simulink model "gm_smartCart4_1_work"  (R2016a)
settings: Solver=FixedStepDiscrete  StartTime=0.0  StopTime=100000  FixedStep=1  RelTol=1e-3
libraries: simulink x103, hdlsllib x73
(part 3 of 3)

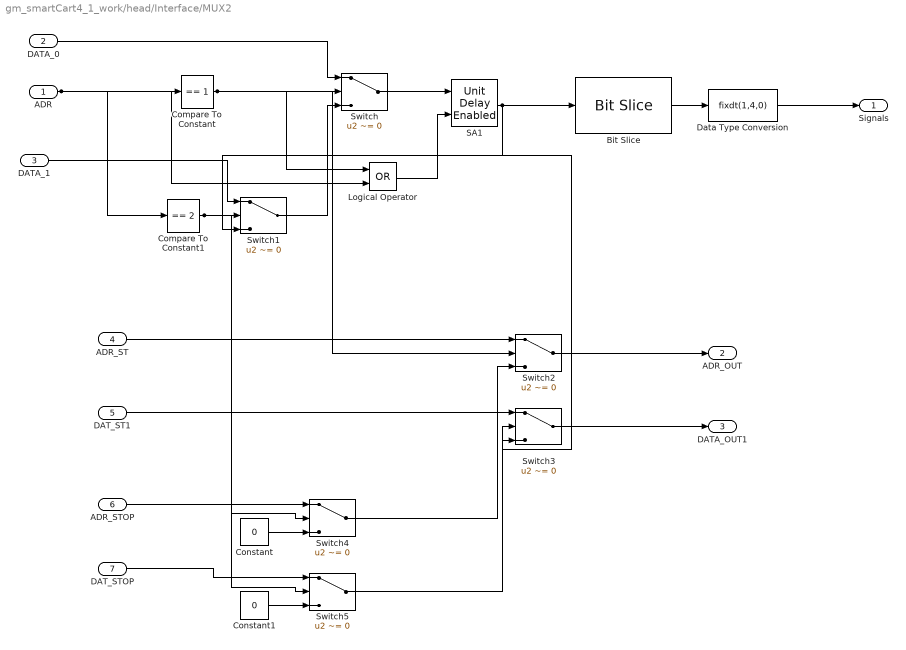
== system gm_smartCart4_1_work/head/Interface/MUX2 ==
  ADR : Inport  OutDataTypeStr=uint8  SampleTime=1
  DATA_0 : Inport  Port=2  OutDataTypeStr=uint8  SampleTime=1
  DATA_1 : Inport  Port=3  OutDataTypeStr=uint8  SampleTime=1
  ADR_ST : Inport  Port=4  OutDataTypeStr=uint8  SampleTime=1
  DAT_ST1 : Inport  Port=5  OutDataTypeStr=uint8  SampleTime=1
  ADR_STOP : Inport  Port=6  OutDataTypeStr=uint8  SampleTime=1
  DAT_STOP : Inport  Port=7  OutDataTypeStr=uint8  SampleTime=1
  Bit Slice : hdlsllib/HDL Operations/Bit Slice  lidx=4  ridx=0
  Compare To Constant : simulink/Logic and Bit Operations/Compare To Constant  relop===  const=1  OutDataTypeStr=boolean
  Compare To Constant1 : simulink/Logic and Bit Operations/Compare To Constant  relop===  const=2  OutDataTypeStr=boolean
  Constant : Constant  Value=0  OutDataTypeStr=boolean
  Constant1 : Constant  Value=0  OutDataTypeStr=boolean
  Data Type Conversion : DataTypeConversion  OutDataTypeStr=fixdt(1,4,0)
  Logical Operator : Logic  Operator=OR  AllPortsSameDT=off  OutDataTypeStr=boolean
  SA1 : simulink/Additional Math & Discrete/Additional Discrete/Unit Delay Enabled  vinit=0  tsamp=-1
  Switch{,1..5} (6 alike) : Switch  Criteria=u2 ~= 0  OutDataTypeStr=uint8
  Signals : Outport  OutDataTypeStr=fixdt(1,4,0)
  ADR_OUT : Outport  Port=2  OutDataTypeStr=uint8
  DATA_OUT1 : Outport  Port=3  OutDataTypeStr=uint8
  wires:
  ADR/1 -> Logical Operator/2, Compare To Constant1/1, Compare To Constant/1
  DATA_0/1 -> Switch/1
  DATA_1/1 -> Switch1/1
  ADR_ST/1 -> Switch2/1
  DAT_ST1/1 -> Switch3/1
  ADR_STOP/1 -> Switch4/1
  DAT_STOP/1 -> Switch5/1
  Bit Slice/1 -> Data Type Conversion/1
  Compare To Constant/1 -> Switch3/2, Switch2/2, Switch/2, Logical Operator/1
  Compare To Constant1/1 -> Switch5/2, Switch4/2, Switch1/2
  Constant/1 -> Switch4/3
  Constant1/1 -> Switch5/3
  Data Type Conversion/1 -> Signals/1
  Logical Operator/1 -> SA1/2
  SA1/1 -> Switch1/3, Bit Slice/1
  Switch/1 -> SA1/1
  Switch1/1 -> Switch/3
  Switch2/1 -> ADR_OUT/1
  Switch3/1 -> DATA_OUT1/1
  Switch4/1 -> Switch2/3
  Switch5/1 -> Switch3/3

== system gm_smartCart4_1_work/head/Interface/Swith_signal2 ==
  Adr : Inport  OutDataTypeStr=uint8  SampleTime=1
  Data : Inport  Port=2  OutDataTypeStr=uint8  SampleTime=1
  Compare To Constant : simulink/Logic and Bit Operations/Compare To Constant  relop===  const=2  OutDataTypeStr=boolean
  SA1 : simulink/Additional Math & Discrete/Additional Discrete/Unit Delay Enabled  vinit=0  tsamp=-1
  OutAddr : Outport  OutDataTypeStr=uint8
  wires:
  Adr/1 -> Compare To Constant/1
  Data/1 -> SA1/1
  Compare To Constant/1 -> SA1/2
  SA1/1 -> OutAddr/1

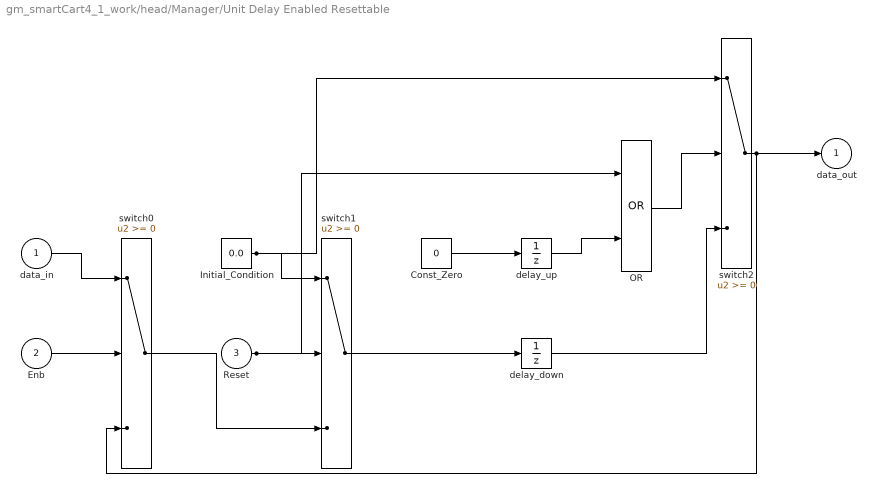
== system gm_smartCart4_1_work/head/Manager/Unit Delay Enabled Resettable ==
  data_in : Inport
  Enb : Inport  Port=2
  Reset : Inport  Port=3
  Const_Zero : Constant  Value=0  OutDataTypeStr=boolean
  Initial_Condition : Constant  Value=0.0  OutDataTypeStr=Inherit: Inherit via back propagation
  OR : Logic  Operator=OR
  delay_down : UnitDelay  SampleTime=-1
  delay_up : UnitDelay  InitialCondition=1  SampleTime=-1
  switch0 : Switch  SaturateOnIntegerOverflow=on  InputSameDT=on
  switch1 : Switch  SaturateOnIntegerOverflow=on  InputSameDT=on
  switch2 : Switch  SaturateOnIntegerOverflow=on  InputSameDT=on
  data_out : Outport
  wires:
  data_in/1 -> switch0/1
  Enb/1 -> switch0/2
  switch2/1 -> switch0/3, data_out/1
  Initial_Condition/1 -> switch1/1, switch2/1
  Reset/1 -> switch1/2, OR/1
  switch0/1 -> switch1/3
  Const_Zero/1 -> delay_up/1
  switch1/1 -> delay_down/1
  delay_up/1 -> OR/2
  OR/1 -> switch2/2
  delay_down/1 -> switch2/3

== system gm_smartCart4_1_work/head/Manager/Unit Delay Enabled Resettable1 ==
  data_in : Inport
  Enb : Inport  Port=2
  Reset : Inport  Port=3
  Const_Zero : Constant  Value=0  OutDataTypeStr=boolean
  Initial_Condition : Constant  Value=0.0  OutDataTypeStr=Inherit: Inherit via back propagation
  OR : Logic  Operator=OR
  delay_down : UnitDelay  SampleTime=-1
  delay_up : UnitDelay  InitialCondition=1  SampleTime=-1
  switch0 : Switch  SaturateOnIntegerOverflow=on  InputSameDT=on
  switch1 : Switch  SaturateOnIntegerOverflow=on  InputSameDT=on
  switch2 : Switch  SaturateOnIntegerOverflow=on  InputSameDT=on
  data_out : Outport
  wires:
  data_in/1 -> switch0/1
  Enb/1 -> switch0/2
  switch2/1 -> switch0/3, data_out/1
  Initial_Condition/1 -> switch1/1, switch2/1
  Reset/1 -> switch1/2, OR/1
  switch0/1 -> switch1/3
  Const_Zero/1 -> delay_up/1
  switch1/1 -> delay_down/1
  delay_up/1 -> OR/2
  OR/1 -> switch2/2
  delay_down/1 -> switch2/3

== system gm_smartCart4_1_work/head/Manager/Unit Delay Enabled Resettable10 ==
  data_in : Inport
  Enb : Inport  Port=2
  Reset : Inport  Port=3
  Const_Zero : Constant  Value=0  OutDataTypeStr=boolean
  Initial_Condition : Constant  Value=0.0  OutDataTypeStr=Inherit: Inherit via back propagation
  OR : Logic  Operator=OR
  delay_down : UnitDelay  SampleTime=-1
  delay_up : UnitDelay  InitialCondition=1  SampleTime=-1
  switch0 : Switch  SaturateOnIntegerOverflow=on  InputSameDT=on
  switch1 : Switch  SaturateOnIntegerOverflow=on  InputSameDT=on
  switch2 : Switch  SaturateOnIntegerOverflow=on  InputSameDT=on
  data_out : Outport
  wires:
  data_in/1 -> switch0/1
  Enb/1 -> switch0/2
  switch2/1 -> switch0/3, data_out/1
  Initial_Condition/1 -> switch1/1, switch2/1
  Reset/1 -> switch1/2, OR/1
  switch0/1 -> switch1/3
  Const_Zero/1 -> delay_up/1
  switch1/1 -> delay_down/1
  delay_up/1 -> OR/2
  OR/1 -> switch2/2
  delay_down/1 -> switch2/3

== system gm_smartCart4_1_work/head/Manager/Unit Delay Enabled Resettable11 ==
  data_in : Inport
  Enb : Inport  Port=2
  Reset : Inport  Port=3
  Const_Zero : Constant  Value=0  OutDataTypeStr=boolean
  Initial_Condition : Constant  Value=0.0  OutDataTypeStr=Inherit: Inherit via back propagation
  OR : Logic  Operator=OR
  delay_down : UnitDelay  SampleTime=-1
  delay_up : UnitDelay  InitialCondition=1  SampleTime=-1
  switch0 : Switch  SaturateOnIntegerOverflow=on  InputSameDT=on
  switch1 : Switch  SaturateOnIntegerOverflow=on  InputSameDT=on
  switch2 : Switch  SaturateOnIntegerOverflow=on  InputSameDT=on
  data_out : Outport
  wires:
  data_in/1 -> switch0/1
  Enb/1 -> switch0/2
  switch2/1 -> switch0/3, data_out/1
  Initial_Condition/1 -> switch1/1, switch2/1
  Reset/1 -> switch1/2, OR/1
  switch0/1 -> switch1/3
  Const_Zero/1 -> delay_up/1
  switch1/1 -> delay_down/1
  delay_up/1 -> OR/2
  OR/1 -> switch2/2
  delay_down/1 -> switch2/3

== system gm_smartCart4_1_work/head/Manager/Unit Delay Enabled Resettable12 ==
  data_in : Inport
  Enb : Inport  Port=2
  Reset : Inport  Port=3
  Const_Zero : Constant  Value=0  OutDataTypeStr=boolean
  Initial_Condition : Constant  Value=0.0  OutDataTypeStr=Inherit: Inherit via back propagation
  OR : Logic  Operator=OR
  delay_down : UnitDelay  SampleTime=-1
  delay_up : UnitDelay  InitialCondition=1  SampleTime=-1
  switch0 : Switch  SaturateOnIntegerOverflow=on  InputSameDT=on
  switch1 : Switch  SaturateOnIntegerOverflow=on  InputSameDT=on
  switch2 : Switch  SaturateOnIntegerOverflow=on  InputSameDT=on
  data_out : Outport
  wires:
  data_in/1 -> switch0/1
  Enb/1 -> switch0/2
  switch2/1 -> switch0/3, data_out/1
  Initial_Condition/1 -> switch1/1, switch2/1
  Reset/1 -> switch1/2, OR/1
  switch0/1 -> switch1/3
  Const_Zero/1 -> delay_up/1
  switch1/1 -> delay_down/1
  delay_up/1 -> OR/2
  OR/1 -> switch2/2
  delay_down/1 -> switch2/3

== system gm_smartCart4_1_work/head/Manager/Unit Delay Enabled Resettable13 ==
  data_in : Inport
  Enb : Inport  Port=2
  Reset : Inport  Port=3
  Const_Zero : Constant  Value=0  OutDataTypeStr=boolean
  Initial_Condition : Constant  Value=0.0  OutDataTypeStr=Inherit: Inherit via back propagation
  OR : Logic  Operator=OR
  delay_down : UnitDelay  SampleTime=-1
  delay_up : UnitDelay  InitialCondition=1  SampleTime=-1
  switch0 : Switch  SaturateOnIntegerOverflow=on  InputSameDT=on
  switch1 : Switch  SaturateOnIntegerOverflow=on  InputSameDT=on
  switch2 : Switch  SaturateOnIntegerOverflow=on  InputSameDT=on
  data_out : Outport
  wires:
  data_in/1 -> switch0/1
  Enb/1 -> switch0/2
  switch2/1 -> switch0/3, data_out/1
  Initial_Condition/1 -> switch1/1, switch2/1
  Reset/1 -> switch1/2, OR/1
  switch0/1 -> switch1/3
  Const_Zero/1 -> delay_up/1
  switch1/1 -> delay_down/1
  delay_up/1 -> OR/2
  OR/1 -> switch2/2
  delay_down/1 -> switch2/3

== system gm_smartCart4_1_work/head/Manager/Unit Delay Enabled Resettable14 ==
  data_in : Inport
  Enb : Inport  Port=2
  Reset : Inport  Port=3
  Const_Zero : Constant  Value=0  OutDataTypeStr=boolean
  Initial_Condition : Constant  Value=0  OutDataTypeStr=Inherit: Inherit via back propagation
  OR : Logic  Operator=OR
  delay_down : UnitDelay  SampleTime=-1
  delay_up : UnitDelay  InitialCondition=1  SampleTime=-1
  switch0 : Switch  SaturateOnIntegerOverflow=on  InputSameDT=on
  switch1 : Switch  SaturateOnIntegerOverflow=on  InputSameDT=on
  switch2 : Switch  SaturateOnIntegerOverflow=on  InputSameDT=on
  data_out : Outport
  wires:
  data_in/1 -> switch0/1
  Enb/1 -> switch0/2
  switch2/1 -> switch0/3, data_out/1
  Initial_Condition/1 -> switch1/1, switch2/1
  Reset/1 -> switch1/2, OR/1
  switch0/1 -> switch1/3
  Const_Zero/1 -> delay_up/1
  switch1/1 -> delay_down/1
  delay_up/1 -> OR/2
  OR/1 -> switch2/2
  delay_down/1 -> switch2/3

== system gm_smartCart4_1_work/head/Manager/Unit Delay Enabled Resettable15 ==
  data_in : Inport
  Enb : Inport  Port=2
  Reset : Inport  Port=3
  Const_Zero : Constant  Value=0  OutDataTypeStr=boolean
  Initial_Condition : Constant  Value=0.0  OutDataTypeStr=Inherit: Inherit via back propagation
  OR : Logic  Operator=OR
  delay_down : UnitDelay  SampleTime=-1
  delay_up : UnitDelay  InitialCondition=1  SampleTime=-1
  switch0 : Switch  SaturateOnIntegerOverflow=on  InputSameDT=on
  switch1 : Switch  SaturateOnIntegerOverflow=on  InputSameDT=on
  switch2 : Switch  SaturateOnIntegerOverflow=on  InputSameDT=on
  data_out : Outport
  wires:
  data_in/1 -> switch0/1
  Enb/1 -> switch0/2
  switch2/1 -> switch0/3, data_out/1
  Initial_Condition/1 -> switch1/1, switch2/1
  Reset/1 -> switch1/2, OR/1
  switch0/1 -> switch1/3
  Const_Zero/1 -> delay_up/1
  switch1/1 -> delay_down/1
  delay_up/1 -> OR/2
  OR/1 -> switch2/2
  delay_down/1 -> switch2/3

== system gm_smartCart4_1_work/head/Manager/Unit Delay Enabled Resettable16 ==
  data_in : Inport
  Enb : Inport  Port=2
  Reset : Inport  Port=3
  Const_Zero : Constant  Value=0  OutDataTypeStr=boolean
  Initial_Condition : Constant  Value=0  OutDataTypeStr=Inherit: Inherit via back propagation
  OR : Logic  Operator=OR
  delay_down : UnitDelay  SampleTime=-1
  delay_up : UnitDelay  InitialCondition=1  SampleTime=-1
  switch0 : Switch  SaturateOnIntegerOverflow=on  InputSameDT=on
  switch1 : Switch  SaturateOnIntegerOverflow=on  InputSameDT=on
  switch2 : Switch  SaturateOnIntegerOverflow=on  InputSameDT=on
  data_out : Outport
  wires:
  data_in/1 -> switch0/1
  Enb/1 -> switch0/2
  switch2/1 -> switch0/3, data_out/1
  Initial_Condition/1 -> switch1/1, switch2/1
  Reset/1 -> switch1/2, OR/1
  switch0/1 -> switch1/3
  Const_Zero/1 -> delay_up/1
  switch1/1 -> delay_down/1
  delay_up/1 -> OR/2
  OR/1 -> switch2/2
  delay_down/1 -> switch2/3

== system gm_smartCart4_1_work/head/Manager/Unit Delay Enabled Resettable17 ==
  data_in : Inport
  Enb : Inport  Port=2
  Reset : Inport  Port=3
  Const_Zero : Constant  Value=0  OutDataTypeStr=boolean
  Initial_Condition : Constant  Value=0  OutDataTypeStr=Inherit: Inherit via back propagation
  OR : Logic  Operator=OR
  delay_down : UnitDelay  SampleTime=-1
  delay_up : UnitDelay  InitialCondition=1  SampleTime=-1
  switch0 : Switch  SaturateOnIntegerOverflow=on  InputSameDT=on
  switch1 : Switch  SaturateOnIntegerOverflow=on  InputSameDT=on
  switch2 : Switch  SaturateOnIntegerOverflow=on  InputSameDT=on
  data_out : Outport
  wires:
  data_in/1 -> switch0/1
  Enb/1 -> switch0/2
  switch2/1 -> switch0/3, data_out/1
  Initial_Condition/1 -> switch1/1, switch2/1
  Reset/1 -> switch1/2, OR/1
  switch0/1 -> switch1/3
  Const_Zero/1 -> delay_up/1
  switch1/1 -> delay_down/1
  delay_up/1 -> OR/2
  OR/1 -> switch2/2
  delay_down/1 -> switch2/3

== system gm_smartCart4_1_work/head/Manager/Unit Delay Enabled Resettable18 ==
  data_in : Inport
  Enb : Inport  Port=2
  Reset : Inport  Port=3
  Const_Zero : Constant  Value=0  OutDataTypeStr=boolean
  Initial_Condition : Constant  Value=0  OutDataTypeStr=Inherit: Inherit via back propagation
  OR : Logic  Operator=OR
  delay_down : UnitDelay  SampleTime=-1
  delay_up : UnitDelay  InitialCondition=1  SampleTime=-1
  switch0 : Switch  SaturateOnIntegerOverflow=on  InputSameDT=on
  switch1 : Switch  SaturateOnIntegerOverflow=on  InputSameDT=on
  switch2 : Switch  SaturateOnIntegerOverflow=on  InputSameDT=on
  data_out : Outport
  wires:
  data_in/1 -> switch0/1
  Enb/1 -> switch0/2
  switch2/1 -> switch0/3, data_out/1
  Initial_Condition/1 -> switch1/1, switch2/1
  Reset/1 -> switch1/2, OR/1
  switch0/1 -> switch1/3
  Const_Zero/1 -> delay_up/1
  switch1/1 -> delay_down/1
  delay_up/1 -> OR/2
  OR/1 -> switch2/2
  delay_down/1 -> switch2/3

== system gm_smartCart4_1_work/head/Manager/Unit Delay Enabled Resettable19 ==
  data_in : Inport
  Enb : Inport  Port=2
  Reset : Inport  Port=3
  Const_Zero : Constant  Value=0  OutDataTypeStr=boolean
  Initial_Condition : Constant  Value=0  OutDataTypeStr=Inherit: Inherit via back propagation
  OR : Logic  Operator=OR
  delay_down : UnitDelay  SampleTime=-1
  delay_up : UnitDelay  InitialCondition=1  SampleTime=-1
  switch0 : Switch  SaturateOnIntegerOverflow=on  InputSameDT=on
  switch1 : Switch  SaturateOnIntegerOverflow=on  InputSameDT=on
  switch2 : Switch  SaturateOnIntegerOverflow=on  InputSameDT=on
  data_out : Outport
  wires:
  data_in/1 -> switch0/1
  Enb/1 -> switch0/2
  switch2/1 -> switch0/3, data_out/1
  Initial_Condition/1 -> switch1/1, switch2/1
  Reset/1 -> switch1/2, OR/1
  switch0/1 -> switch1/3
  Const_Zero/1 -> delay_up/1
  switch1/1 -> delay_down/1
  delay_up/1 -> OR/2
  OR/1 -> switch2/2
  delay_down/1 -> switch2/3

== system gm_smartCart4_1_work/head/Manager/Unit Delay Enabled Resettable2 ==
  data_in : Inport
  Enb : Inport  Port=2
  Reset : Inport  Port=3
  Const_Zero : Constant  Value=0  OutDataTypeStr=boolean
  Initial_Condition : Constant  Value=0.0  OutDataTypeStr=Inherit: Inherit via back propagation
  OR : Logic  Operator=OR
  delay_down : UnitDelay  SampleTime=-1
  delay_up : UnitDelay  InitialCondition=1  SampleTime=-1
  switch0 : Switch  SaturateOnIntegerOverflow=on  InputSameDT=on
  switch1 : Switch  SaturateOnIntegerOverflow=on  InputSameDT=on
  switch2 : Switch  SaturateOnIntegerOverflow=on  InputSameDT=on
  data_out : Outport
  wires:
  data_in/1 -> switch0/1
  Enb/1 -> switch0/2
  switch2/1 -> switch0/3, data_out/1
  Initial_Condition/1 -> switch1/1, switch2/1
  Reset/1 -> switch1/2, OR/1
  switch0/1 -> switch1/3
  Const_Zero/1 -> delay_up/1
  switch1/1 -> delay_down/1
  delay_up/1 -> OR/2
  OR/1 -> switch2/2
  delay_down/1 -> switch2/3

== system gm_smartCart4_1_work/head/Manager/Unit Delay Enabled Resettable20 ==
  data_in : Inport
  Enb : Inport  Port=2
  Reset : Inport  Port=3
  Const_Zero : Constant  Value=0  OutDataTypeStr=boolean
  Initial_Condition : Constant  Value=0  OutDataTypeStr=Inherit: Inherit via back propagation
  OR : Logic  Operator=OR
  delay_down : UnitDelay  SampleTime=-1
  delay_up : UnitDelay  InitialCondition=1  SampleTime=-1
  switch0 : Switch  SaturateOnIntegerOverflow=on  InputSameDT=on
  switch1 : Switch  SaturateOnIntegerOverflow=on  InputSameDT=on
  switch2 : Switch  SaturateOnIntegerOverflow=on  InputSameDT=on
  data_out : Outport
  wires:
  data_in/1 -> switch0/1
  Enb/1 -> switch0/2
  switch2/1 -> switch0/3, data_out/1
  Initial_Condition/1 -> switch1/1, switch2/1
  Reset/1 -> switch1/2, OR/1
  switch0/1 -> switch1/3
  Const_Zero/1 -> delay_up/1
  switch1/1 -> delay_down/1
  delay_up/1 -> OR/2
  OR/1 -> switch2/2
  delay_down/1 -> switch2/3

== system gm_smartCart4_1_work/head/Manager/Unit Delay Enabled Resettable21 ==
  data_in : Inport
  Enb : Inport  Port=2
  Reset : Inport  Port=3
  Const_Zero : Constant  Value=0  OutDataTypeStr=boolean
  Initial_Condition : Constant  Value=0  OutDataTypeStr=Inherit: Inherit via back propagation
  OR : Logic  Operator=OR
  delay_down : UnitDelay  SampleTime=-1
  delay_up : UnitDelay  InitialCondition=1  SampleTime=-1
  switch0 : Switch  SaturateOnIntegerOverflow=on  InputSameDT=on
  switch1 : Switch  SaturateOnIntegerOverflow=on  InputSameDT=on
  switch2 : Switch  SaturateOnIntegerOverflow=on  InputSameDT=on
  data_out : Outport
  wires:
  data_in/1 -> switch0/1
  Enb/1 -> switch0/2
  switch2/1 -> switch0/3, data_out/1
  Initial_Condition/1 -> switch1/1, switch2/1
  Reset/1 -> switch1/2, OR/1
  switch0/1 -> switch1/3
  Const_Zero/1 -> delay_up/1
  switch1/1 -> delay_down/1
  delay_up/1 -> OR/2
  OR/1 -> switch2/2
  delay_down/1 -> switch2/3

== system gm_smartCart4_1_work/head/Manager/Unit Delay Enabled Resettable22 ==
  data_in : Inport
  Enb : Inport  Port=2
  Reset : Inport  Port=3
  Const_Zero : Constant  Value=0  OutDataTypeStr=boolean
  Initial_Condition : Constant  Value=0  OutDataTypeStr=Inherit: Inherit via back propagation
  OR : Logic  Operator=OR
  delay_down : UnitDelay  SampleTime=-1
  delay_up : UnitDelay  InitialCondition=1  SampleTime=-1
  switch0 : Switch  SaturateOnIntegerOverflow=on  InputSameDT=on
  switch1 : Switch  SaturateOnIntegerOverflow=on  InputSameDT=on
  switch2 : Switch  SaturateOnIntegerOverflow=on  InputSameDT=on
  data_out : Outport
  wires:
  data_in/1 -> switch0/1
  Enb/1 -> switch0/2
  switch2/1 -> switch0/3, data_out/1
  Initial_Condition/1 -> switch1/1, switch2/1
  Reset/1 -> switch1/2, OR/1
  switch0/1 -> switch1/3
  Const_Zero/1 -> delay_up/1
  switch1/1 -> delay_down/1
  delay_up/1 -> OR/2
  OR/1 -> switch2/2
  delay_down/1 -> switch2/3

== system gm_smartCart4_1_work/head/Manager/Unit Delay Enabled Resettable23 ==
  data_in : Inport
  Enb : Inport  Port=2
  Reset : Inport  Port=3
  Const_Zero : Constant  Value=0  OutDataTypeStr=boolean
  Initial_Condition : Constant  Value=0  OutDataTypeStr=Inherit: Inherit via back propagation
  OR : Logic  Operator=OR
  delay_down : UnitDelay  SampleTime=-1
  delay_up : UnitDelay  InitialCondition=1  SampleTime=-1
  switch0 : Switch  SaturateOnIntegerOverflow=on  InputSameDT=on
  switch1 : Switch  SaturateOnIntegerOverflow=on  InputSameDT=on
  switch2 : Switch  SaturateOnIntegerOverflow=on  InputSameDT=on
  data_out : Outport
  wires:
  data_in/1 -> switch0/1
  Enb/1 -> switch0/2
  switch2/1 -> switch0/3, data_out/1
  Initial_Condition/1 -> switch1/1, switch2/1
  Reset/1 -> switch1/2, OR/1
  switch0/1 -> switch1/3
  Const_Zero/1 -> delay_up/1
  switch1/1 -> delay_down/1
  delay_up/1 -> OR/2
  OR/1 -> switch2/2
  delay_down/1 -> switch2/3

== system gm_smartCart4_1_work/head/Manager/Unit Delay Enabled Resettable24 ==
  data_in : Inport
  Enb : Inport  Port=2
  Reset : Inport  Port=3
  Const_Zero : Constant  Value=0  OutDataTypeStr=boolean
  Initial_Condition : Constant  Value=0  OutDataTypeStr=Inherit: Inherit via back propagation
  OR : Logic  Operator=OR
  delay_down : UnitDelay  SampleTime=-1
  delay_up : UnitDelay  InitialCondition=1  SampleTime=-1
  switch0 : Switch  SaturateOnIntegerOverflow=on  InputSameDT=on
  switch1 : Switch  SaturateOnIntegerOverflow=on  InputSameDT=on
  switch2 : Switch  SaturateOnIntegerOverflow=on  InputSameDT=on
  data_out : Outport
  wires:
  data_in/1 -> switch0/1
  Enb/1 -> switch0/2
  switch2/1 -> switch0/3, data_out/1
  Initial_Condition/1 -> switch1/1, switch2/1
  Reset/1 -> switch1/2, OR/1
  switch0/1 -> switch1/3
  Const_Zero/1 -> delay_up/1
  switch1/1 -> delay_down/1
  delay_up/1 -> OR/2
  OR/1 -> switch2/2
  delay_down/1 -> switch2/3

== system gm_smartCart4_1_work/head/Manager/Unit Delay Enabled Resettable26 ==
  data_in : Inport
  Enb : Inport  Port=2
  Reset : Inport  Port=3
  Const_Zero : Constant  Value=0  OutDataTypeStr=boolean
  Initial_Condition : Constant  Value=0  OutDataTypeStr=Inherit: Inherit via back propagation
  OR : Logic  Operator=OR
  delay_down : UnitDelay  SampleTime=-1
  delay_up : UnitDelay  InitialCondition=1  SampleTime=-1
  switch0 : Switch  SaturateOnIntegerOverflow=on  InputSameDT=on
  switch1 : Switch  SaturateOnIntegerOverflow=on  InputSameDT=on
  switch2 : Switch  SaturateOnIntegerOverflow=on  InputSameDT=on
  data_out : Outport
  wires:
  data_in/1 -> switch0/1
  Enb/1 -> switch0/2
  switch2/1 -> switch0/3, data_out/1
  Initial_Condition/1 -> switch1/1, switch2/1
  Reset/1 -> switch1/2, OR/1
  switch0/1 -> switch1/3
  Const_Zero/1 -> delay_up/1
  switch1/1 -> delay_down/1
  delay_up/1 -> OR/2
  OR/1 -> switch2/2
  delay_down/1 -> switch2/3

== system gm_smartCart4_1_work/head/Manager/Unit Delay Enabled Resettable28 ==
  data_in : Inport
  Enb : Inport  Port=2
  Reset : Inport  Port=3
  Const_Zero : Constant  Value=0  OutDataTypeStr=boolean
  Initial_Condition : Constant  Value=0  OutDataTypeStr=Inherit: Inherit via back propagation
  OR : Logic  Operator=OR
  delay_down : UnitDelay  SampleTime=-1
  delay_up : UnitDelay  InitialCondition=1  SampleTime=-1
  switch0 : Switch  SaturateOnIntegerOverflow=on  InputSameDT=on
  switch1 : Switch  SaturateOnIntegerOverflow=on  InputSameDT=on
  switch2 : Switch  SaturateOnIntegerOverflow=on  InputSameDT=on
  data_out : Outport
  wires:
  data_in/1 -> switch0/1
  Enb/1 -> switch0/2
  switch2/1 -> switch0/3, data_out/1
  Initial_Condition/1 -> switch1/1, switch2/1
  Reset/1 -> switch1/2, OR/1
  switch0/1 -> switch1/3
  Const_Zero/1 -> delay_up/1
  switch1/1 -> delay_down/1
  delay_up/1 -> OR/2
  OR/1 -> switch2/2
  delay_down/1 -> switch2/3

== system gm_smartCart4_1_work/head/Manager/Unit Delay Enabled Resettable3 ==
  data_in : Inport
  Enb : Inport  Port=2
  Reset : Inport  Port=3
  Const_Zero : Constant  Value=0  OutDataTypeStr=boolean
  Initial_Condition : Constant  Value=0  OutDataTypeStr=Inherit: Inherit via back propagation
  OR : Logic  Operator=OR
  delay_down : UnitDelay  SampleTime=-1
  delay_up : UnitDelay  InitialCondition=1  SampleTime=-1
  switch0 : Switch  SaturateOnIntegerOverflow=on  InputSameDT=on
  switch1 : Switch  SaturateOnIntegerOverflow=on  InputSameDT=on
  switch2 : Switch  SaturateOnIntegerOverflow=on  InputSameDT=on
  data_out : Outport
  wires:
  data_in/1 -> switch0/1
  Enb/1 -> switch0/2
  switch2/1 -> switch0/3, data_out/1
  Initial_Condition/1 -> switch1/1, switch2/1
  Reset/1 -> switch1/2, OR/1
  switch0/1 -> switch1/3
  Const_Zero/1 -> delay_up/1
  switch1/1 -> delay_down/1
  delay_up/1 -> OR/2
  OR/1 -> switch2/2
  delay_down/1 -> switch2/3

== system gm_smartCart4_1_work/head/Manager/Unit Delay Enabled Resettable4 ==
  data_in : Inport
  Enb : Inport  Port=2
  Reset : Inport  Port=3
  Const_Zero : Constant  Value=0  OutDataTypeStr=boolean
  Initial_Condition : Constant  Value=0  OutDataTypeStr=Inherit: Inherit via back propagation
  OR : Logic  Operator=OR
  delay_down : UnitDelay  SampleTime=-1
  delay_up : UnitDelay  InitialCondition=1  SampleTime=-1
  switch0 : Switch  SaturateOnIntegerOverflow=on  InputSameDT=on
  switch1 : Switch  SaturateOnIntegerOverflow=on  InputSameDT=on
  switch2 : Switch  SaturateOnIntegerOverflow=on  InputSameDT=on
  data_out : Outport
  wires:
  data_in/1 -> switch0/1
  Enb/1 -> switch0/2
  switch2/1 -> switch0/3, data_out/1
  Initial_Condition/1 -> switch1/1, switch2/1
  Reset/1 -> switch1/2, OR/1
  switch0/1 -> switch1/3
  Const_Zero/1 -> delay_up/1
  switch1/1 -> delay_down/1
  delay_up/1 -> OR/2
  OR/1 -> switch2/2
  delay_down/1 -> switch2/3

== system gm_smartCart4_1_work/head/Manager/Unit Delay Enabled Resettable5 ==
  data_in : Inport
  Enb : Inport  Port=2
  Reset : Inport  Port=3
  Const_Zero : Constant  Value=0  OutDataTypeStr=boolean
  Initial_Condition : Constant  Value=0.0  OutDataTypeStr=Inherit: Inherit via back propagation
  OR : Logic  Operator=OR
  delay_down : UnitDelay  SampleTime=-1
  delay_up : UnitDelay  InitialCondition=1  SampleTime=-1
  switch0 : Switch  SaturateOnIntegerOverflow=on  InputSameDT=on
  switch1 : Switch  SaturateOnIntegerOverflow=on  InputSameDT=on
  switch2 : Switch  SaturateOnIntegerOverflow=on  InputSameDT=on
  data_out : Outport
  wires:
  data_in/1 -> switch0/1
  Enb/1 -> switch0/2
  switch2/1 -> switch0/3, data_out/1
  Initial_Condition/1 -> switch1/1, switch2/1
  Reset/1 -> switch1/2, OR/1
  switch0/1 -> switch1/3
  Const_Zero/1 -> delay_up/1
  switch1/1 -> delay_down/1
  delay_up/1 -> OR/2
  OR/1 -> switch2/2
  delay_down/1 -> switch2/3

== system gm_smartCart4_1_work/head/Manager/Unit Delay Enabled Resettable6 ==
  data_in : Inport
  Enb : Inport  Port=2
  Reset : Inport  Port=3
  Const_Zero : Constant  Value=0  OutDataTypeStr=boolean
  Initial_Condition : Constant  Value=0.0  OutDataTypeStr=Inherit: Inherit via back propagation
  OR : Logic  Operator=OR
  delay_down : UnitDelay  SampleTime=-1
  delay_up : UnitDelay  InitialCondition=1  SampleTime=-1
  switch0 : Switch  SaturateOnIntegerOverflow=on  InputSameDT=on
  switch1 : Switch  SaturateOnIntegerOverflow=on  InputSameDT=on
  switch2 : Switch  SaturateOnIntegerOverflow=on  InputSameDT=on
  data_out : Outport
  wires:
  data_in/1 -> switch0/1
  Enb/1 -> switch0/2
  switch2/1 -> switch0/3, data_out/1
  Initial_Condition/1 -> switch1/1, switch2/1
  Reset/1 -> switch1/2, OR/1
  switch0/1 -> switch1/3
  Const_Zero/1 -> delay_up/1
  switch1/1 -> delay_down/1
  delay_up/1 -> OR/2
  OR/1 -> switch2/2
  delay_down/1 -> switch2/3

== system gm_smartCart4_1_work/head/Manager/Unit Delay Enabled Resettable7 ==
  data_in : Inport
  Enb : Inport  Port=2
  Reset : Inport  Port=3
  Const_Zero : Constant  Value=0  OutDataTypeStr=boolean
  Initial_Condition : Constant  Value=0.0  OutDataTypeStr=Inherit: Inherit via back propagation
  OR : Logic  Operator=OR
  delay_down : UnitDelay  SampleTime=-1
  delay_up : UnitDelay  InitialCondition=1  SampleTime=-1
  switch0 : Switch  SaturateOnIntegerOverflow=on  InputSameDT=on
  switch1 : Switch  SaturateOnIntegerOverflow=on  InputSameDT=on
  switch2 : Switch  SaturateOnIntegerOverflow=on  InputSameDT=on
  data_out : Outport
  wires:
  data_in/1 -> switch0/1
  Enb/1 -> switch0/2
  switch2/1 -> switch0/3, data_out/1
  Initial_Condition/1 -> switch1/1, switch2/1
  Reset/1 -> switch1/2, OR/1
  switch0/1 -> switch1/3
  Const_Zero/1 -> delay_up/1
  switch1/1 -> delay_down/1
  delay_up/1 -> OR/2
  OR/1 -> switch2/2
  delay_down/1 -> switch2/3

== system gm_smartCart4_1_work/head/Manager/Unit Delay Enabled Resettable8 ==
  data_in : Inport
  Enb : Inport  Port=2
  Reset : Inport  Port=3
  Const_Zero : Constant  Value=0  OutDataTypeStr=boolean
  Initial_Condition : Constant  Value=0.0  OutDataTypeStr=Inherit: Inherit via back propagation
  OR : Logic  Operator=OR
  delay_down : UnitDelay  SampleTime=-1
  delay_up : UnitDelay  InitialCondition=1  SampleTime=-1
  switch0 : Switch  SaturateOnIntegerOverflow=on  InputSameDT=on
  switch1 : Switch  SaturateOnIntegerOverflow=on  InputSameDT=on
  switch2 : Switch  SaturateOnIntegerOverflow=on  InputSameDT=on
  data_out : Outport
  wires:
  data_in/1 -> switch0/1
  Enb/1 -> switch0/2
  switch2/1 -> switch0/3, data_out/1
  Initial_Condition/1 -> switch1/1, switch2/1
  Reset/1 -> switch1/2, OR/1
  switch0/1 -> switch1/3
  Const_Zero/1 -> delay_up/1
  switch1/1 -> delay_down/1
  delay_up/1 -> OR/2
  OR/1 -> switch2/2
  delay_down/1 -> switch2/3

== system gm_smartCart4_1_work/head/Manager/Unit Delay Enabled Resettable9 ==
  data_in : Inport
  Enb : Inport  Port=2
  Reset : Inport  Port=3
  Const_Zero : Constant  Value=0  OutDataTypeStr=boolean
  Initial_Condition : Constant  Value=0.0  OutDataTypeStr=Inherit: Inherit via back propagation
  OR : Logic  Operator=OR
  delay_down : UnitDelay  SampleTime=-1
  delay_up : UnitDelay  InitialCondition=1  SampleTime=-1
  switch0 : Switch  SaturateOnIntegerOverflow=on  InputSameDT=on
  switch1 : Switch  SaturateOnIntegerOverflow=on  InputSameDT=on
  switch2 : Switch  SaturateOnIntegerOverflow=on  InputSameDT=on
  data_out : Outport
  wires:
  data_in/1 -> switch0/1
  Enb/1 -> switch0/2
  switch2/1 -> switch0/3, data_out/1
  Initial_Condition/1 -> switch1/1, switch2/1
  Reset/1 -> switch1/2, OR/1
  switch0/1 -> switch1/3
  Const_Zero/1 -> delay_up/1
  switch1/1 -> delay_down/1
  delay_up/1 -> OR/2
  OR/1 -> switch2/2
  delay_down/1 -> switch2/3

== system gm_smartCart4_1_work/head/Manager/signal_edg ==
  In1 : Inport  OutDataTypeStr=boolean  SampleTime=1
  Delay4 : Delay  DelayLength=1  InitialCondition=0
  Logical Operator1 : Logic  Operator=XOR  AllPortsSameDT=off  OutDataTypeStr=boolean
  Logical Operator15 : Logic  AllPortsSameDT=off  OutDataTypeStr=boolean
  Out1 : Outport  OutDataTypeStr=boolean
  wires:
  In1/1 -> Logical Operator15/2, Logical Operator1/2, Delay4/1
  Delay4/1 -> Logical Operator1/1
  Logical Operator1/1 -> Logical Operator15/1
  Logical Operator15/1 -> Out1/1

== system gm_smartCart4_1_work/head/Manager/signal_edg1 ==
  In1 : Inport  OutDataTypeStr=boolean  SampleTime=1
  Delay4 : Delay  DelayLength=1  InitialCondition=0
  Logical Operator1 : Logic  Operator=XOR  AllPortsSameDT=off  OutDataTypeStr=boolean
  Logical Operator15 : Logic  AllPortsSameDT=off  OutDataTypeStr=boolean
  Out1 : Outport  OutDataTypeStr=boolean
  wires:
  Logical Operator15/1 -> Out1/1
  Logical Operator1/1 -> Logical Operator15/1
  Delay4/1 -> Logical Operator1/1
  In1/1 -> Delay4/1, Logical Operator1/2, Logical Operator15/2

== system gm_smartCart4_1_work/head/Manager/signal_edg10 ==
  In1 : Inport  OutDataTypeStr=boolean  SampleTime=1
  Delay4 : Delay  DelayLength=1  InitialCondition=0
  Logical Operator1 : Logic  Operator=XOR  AllPortsSameDT=off  OutDataTypeStr=boolean
  Logical Operator15 : Logic  AllPortsSameDT=off  OutDataTypeStr=boolean
  Out1 : Outport  OutDataTypeStr=boolean
  wires:
  Logical Operator15/1 -> Out1/1
  Logical Operator1/1 -> Logical Operator15/1
  Delay4/1 -> Logical Operator1/1
  In1/1 -> Delay4/1, Logical Operator1/2, Logical Operator15/2

== system gm_smartCart4_1_work/head/Manager/signal_edg2 ==
  In1 : Inport  OutDataTypeStr=boolean  SampleTime=1
  Delay4 : Delay  DelayLength=1  InitialCondition=0
  Logical Operator1 : Logic  Operator=XOR  AllPortsSameDT=off  OutDataTypeStr=boolean
  Logical Operator15 : Logic  AllPortsSameDT=off  OutDataTypeStr=boolean
  Out1 : Outport  OutDataTypeStr=boolean
  wires:
  Logical Operator15/1 -> Out1/1
  Logical Operator1/1 -> Logical Operator15/1
  Delay4/1 -> Logical Operator1/1
  In1/1 -> Delay4/1, Logical Operator1/2, Logical Operator15/2

== system gm_smartCart4_1_work/head/Manager/signal_edg3 ==
  In1 : Inport  OutDataTypeStr=boolean  SampleTime=1
  Delay4 : Delay  DelayLength=1  InitialCondition=0
  Logical Operator1 : Logic  Operator=XOR  AllPortsSameDT=off  OutDataTypeStr=boolean
  Logical Operator15 : Logic  AllPortsSameDT=off  OutDataTypeStr=boolean
  Out1 : Outport  OutDataTypeStr=boolean
  wires:
  Logical Operator15/1 -> Out1/1
  Logical Operator1/1 -> Logical Operator15/1
  Delay4/1 -> Logical Operator1/1
  In1/1 -> Delay4/1, Logical Operator1/2, Logical Operator15/2

== system gm_smartCart4_1_work/head/Manager/signal_edg4 ==
  In1 : Inport  OutDataTypeStr=boolean  SampleTime=1
  Delay4 : Delay  DelayLength=1  InitialCondition=0
  Logical Operator1 : Logic  Operator=XOR  AllPortsSameDT=off  OutDataTypeStr=boolean
  Logical Operator15 : Logic  AllPortsSameDT=off  OutDataTypeStr=boolean
  Out1 : Outport  OutDataTypeStr=boolean
  wires:
  Logical Operator15/1 -> Out1/1
  Logical Operator1/1 -> Logical Operator15/1
  Delay4/1 -> Logical Operator1/1
  In1/1 -> Delay4/1, Logical Operator1/2, Logical Operator15/2

== system gm_smartCart4_1_work/head/Manager/signal_edg5 ==
  In1 : Inport  OutDataTypeStr=boolean  SampleTime=1
  Delay4 : Delay  DelayLength=1  InitialCondition=0
  Logical Operator1 : Logic  Operator=XOR  AllPortsSameDT=off  OutDataTypeStr=boolean
  Logical Operator15 : Logic  AllPortsSameDT=off  OutDataTypeStr=boolean
  Out1 : Outport  OutDataTypeStr=boolean
  wires:
  Logical Operator15/1 -> Out1/1
  Logical Operator1/1 -> Logical Operator15/1
  Delay4/1 -> Logical Operator1/1
  In1/1 -> Delay4/1, Logical Operator1/2, Logical Operator15/2

== system gm_smartCart4_1_work/head/Manager/signal_edg6 ==
  In1 : Inport  OutDataTypeStr=boolean  SampleTime=1
  Delay4 : Delay  DelayLength=1  InitialCondition=0
  Logical Operator1 : Logic  Operator=XOR  AllPortsSameDT=off  OutDataTypeStr=boolean
  Logical Operator15 : Logic  AllPortsSameDT=off  OutDataTypeStr=boolean
  Out1 : Outport  OutDataTypeStr=boolean
  wires:
  Logical Operator15/1 -> Out1/1
  Logical Operator1/1 -> Logical Operator15/1
  Delay4/1 -> Logical Operator1/1
  In1/1 -> Delay4/1, Logical Operator1/2, Logical Operator15/2

== system gm_smartCart4_1_work/head/Manager/signal_edg7 ==
  In1 : Inport  OutDataTypeStr=boolean  SampleTime=1
  Delay4 : Delay  DelayLength=1  InitialCondition=0
  Logical Operator1 : Logic  Operator=XOR  AllPortsSameDT=off  OutDataTypeStr=boolean
  Logical Operator15 : Logic  AllPortsSameDT=off  OutDataTypeStr=boolean
  Out1 : Outport  OutDataTypeStr=boolean
  wires:
  Logical Operator15/1 -> Out1/1
  Logical Operator1/1 -> Logical Operator15/1
  Delay4/1 -> Logical Operator1/1
  In1/1 -> Delay4/1, Logical Operator1/2, Logical Operator15/2

== system gm_smartCart4_1_work/head/Manager/signal_edg8 ==
  In1 : Inport  OutDataTypeStr=boolean  SampleTime=1
  Delay4 : Delay  DelayLength=1  InitialCondition=0
  Logical Operator1 : Logic  Operator=XOR  AllPortsSameDT=off  OutDataTypeStr=boolean
  Logical Operator15 : Logic  AllPortsSameDT=off  OutDataTypeStr=boolean
  Out1 : Outport  OutDataTypeStr=boolean
  wires:
  Logical Operator15/1 -> Out1/1
  Logical Operator1/1 -> Logical Operator15/1
  Delay4/1 -> Logical Operator1/1
  In1/1 -> Delay4/1, Logical Operator1/2, Logical Operator15/2

== system gm_smartCart4_1_work/head/Manager/signal_edg9 ==
  In1 : Inport  OutDataTypeStr=boolean  SampleTime=1
  Delay4 : Delay  DelayLength=1  InitialCondition=0
  Logical Operator1 : Logic  Operator=XOR  AllPortsSameDT=off  OutDataTypeStr=boolean
  Logical Operator15 : Logic  AllPortsSameDT=off  OutDataTypeStr=boolean
  Out1 : Outport  OutDataTypeStr=boolean
  wires:
  Logical Operator15/1 -> Out1/1
  Logical Operator1/1 -> Logical Operator15/1
  Delay4/1 -> Logical Operator1/1
  In1/1 -> Delay4/1, Logical Operator1/2, Logical Operator15/2

== system gm_smartCart4_1_work/head/Reciver/Unit Delay Enabled Resettable ==
  data_in : Inport
  Enb : Inport  Port=2
  Reset : Inport  Port=3
  Const_Zero : Constant  Value=0  OutDataTypeStr=boolean
  Initial_Condition : Constant  Value=0.0  OutDataTypeStr=Inherit: Inherit via back propagation
  OR : Logic  Operator=OR
  delay_down : UnitDelay  SampleTime=-1
  delay_up : UnitDelay  InitialCondition=1  SampleTime=-1
  switch0 : Switch  SaturateOnIntegerOverflow=on  InputSameDT=on
  switch1 : Switch  SaturateOnIntegerOverflow=on  InputSameDT=on
  switch2 : Switch  SaturateOnIntegerOverflow=on  InputSameDT=on
  data_out : Outport
  wires:
  data_in/1 -> switch0/1
  Enb/1 -> switch0/2
  switch2/1 -> switch0/3, data_out/1
  Initial_Condition/1 -> switch1/1, switch2/1
  Reset/1 -> switch1/2, OR/1
  switch0/1 -> switch1/3
  Const_Zero/1 -> delay_up/1
  switch1/1 -> delay_down/1
  delay_up/1 -> OR/2
  OR/1 -> switch2/2
  delay_down/1 -> switch2/3

== system gm_smartCart4_1_work/head/Reciver/Unit Delay Enabled Resettable1 ==
  data_in : Inport
  Enb : Inport  Port=2
  Reset : Inport  Port=3
  Const_Zero : Constant  Value=0  OutDataTypeStr=boolean
  Initial_Condition : Constant  Value=0.0  OutDataTypeStr=Inherit: Inherit via back propagation
  OR : Logic  Operator=OR
  delay_down : UnitDelay  SampleTime=-1
  delay_up : UnitDelay  InitialCondition=1  SampleTime=-1
  switch0 : Switch  SaturateOnIntegerOverflow=on  InputSameDT=on
  switch1 : Switch  SaturateOnIntegerOverflow=on  InputSameDT=on
  switch2 : Switch  SaturateOnIntegerOverflow=on  InputSameDT=on
  data_out : Outport
  wires:
  data_in/1 -> switch0/1
  Enb/1 -> switch0/2
  switch2/1 -> switch0/3, data_out/1
  Initial_Condition/1 -> switch1/1, switch2/1
  Reset/1 -> switch1/2, OR/1
  switch0/1 -> switch1/3
  Const_Zero/1 -> delay_up/1
  switch1/1 -> delay_down/1
  delay_up/1 -> OR/2
  OR/1 -> switch2/2
  delay_down/1 -> switch2/3

== system gm_smartCart4_1_work/head/Reciver/Unit Delay Enabled Resettable11 ==
  data_in : Inport
  Enb : Inport  Port=2
  Reset : Inport  Port=3
  Const_Zero : Constant  Value=0  OutDataTypeStr=boolean
  Initial_Condition : Constant  Value=0.0  OutDataTypeStr=Inherit: Inherit via back propagation
  OR : Logic  Operator=OR
  delay_down : UnitDelay  SampleTime=-1
  delay_up : UnitDelay  InitialCondition=1  SampleTime=-1
  switch0 : Switch  SaturateOnIntegerOverflow=on  InputSameDT=on
  switch1 : Switch  SaturateOnIntegerOverflow=on  InputSameDT=on
  switch2 : Switch  SaturateOnIntegerOverflow=on  InputSameDT=on
  data_out : Outport
  wires:
  data_in/1 -> switch0/1
  Enb/1 -> switch0/2
  switch2/1 -> switch0/3, data_out/1
  Initial_Condition/1 -> switch1/1, switch2/1
  Reset/1 -> switch1/2, OR/1
  switch0/1 -> switch1/3
  Const_Zero/1 -> delay_up/1
  switch1/1 -> delay_down/1
  delay_up/1 -> OR/2
  OR/1 -> switch2/2
  delay_down/1 -> switch2/3

== system gm_smartCart4_1_work/head/Reciver/Unit Delay Enabled Resettable12 ==
  data_in : Inport
  Enb : Inport  Port=2
  Reset : Inport  Port=3
  Const_Zero : Constant  Value=0  OutDataTypeStr=boolean
  Initial_Condition : Constant  Value=0.0  OutDataTypeStr=Inherit: Inherit via back propagation
  OR : Logic  Operator=OR
  delay_down : UnitDelay  SampleTime=-1
  delay_up : UnitDelay  InitialCondition=1  SampleTime=-1
  switch0 : Switch  SaturateOnIntegerOverflow=on  InputSameDT=on
  switch1 : Switch  SaturateOnIntegerOverflow=on  InputSameDT=on
  switch2 : Switch  SaturateOnIntegerOverflow=on  InputSameDT=on
  data_out : Outport
  wires:
  data_in/1 -> switch0/1
  Enb/1 -> switch0/2
  switch2/1 -> switch0/3, data_out/1
  Initial_Condition/1 -> switch1/1, switch2/1
  Reset/1 -> switch1/2, OR/1
  switch0/1 -> switch1/3
  Const_Zero/1 -> delay_up/1
  switch1/1 -> delay_down/1
  delay_up/1 -> OR/2
  OR/1 -> switch2/2
  delay_down/1 -> switch2/3

== system gm_smartCart4_1_work/head/Reciver/Unit Delay Enabled Resettable13 ==
  data_in : Inport
  Enb : Inport  Port=2
  Reset : Inport  Port=3
  Const_Zero : Constant  Value=0  OutDataTypeStr=boolean
  Initial_Condition : Constant  Value=0.0  OutDataTypeStr=Inherit: Inherit via back propagation
  OR : Logic  Operator=OR
  delay_down : UnitDelay  SampleTime=-1
  delay_up : UnitDelay  InitialCondition=1  SampleTime=-1
  switch0 : Switch  SaturateOnIntegerOverflow=on  InputSameDT=on
  switch1 : Switch  SaturateOnIntegerOverflow=on  InputSameDT=on
  switch2 : Switch  SaturateOnIntegerOverflow=on  InputSameDT=on
  data_out : Outport
  wires:
  data_in/1 -> switch0/1
  Enb/1 -> switch0/2
  switch2/1 -> switch0/3, data_out/1
  Initial_Condition/1 -> switch1/1, switch2/1
  Reset/1 -> switch1/2, OR/1
  switch0/1 -> switch1/3
  Const_Zero/1 -> delay_up/1
  switch1/1 -> delay_down/1
  delay_up/1 -> OR/2
  OR/1 -> switch2/2
  delay_down/1 -> switch2/3

== system gm_smartCart4_1_work/head/Reciver/Unit Delay Enabled Resettable14 ==
  data_in : Inport
  Enb : Inport  Port=2
  Reset : Inport  Port=3
  Const_Zero : Constant  Value=0  OutDataTypeStr=boolean
  Initial_Condition : Constant  Value=0.0  OutDataTypeStr=Inherit: Inherit via back propagation
  OR : Logic  Operator=OR
  delay_down : UnitDelay  SampleTime=-1
  delay_up : UnitDelay  InitialCondition=1  SampleTime=-1
  switch0 : Switch  SaturateOnIntegerOverflow=on  InputSameDT=on
  switch1 : Switch  SaturateOnIntegerOverflow=on  InputSameDT=on
  switch2 : Switch  SaturateOnIntegerOverflow=on  InputSameDT=on
  data_out : Outport
  wires:
  data_in/1 -> switch0/1
  Enb/1 -> switch0/2
  switch2/1 -> switch0/3, data_out/1
  Initial_Condition/1 -> switch1/1, switch2/1
  Reset/1 -> switch1/2, OR/1
  switch0/1 -> switch1/3
  Const_Zero/1 -> delay_up/1
  switch1/1 -> delay_down/1
  delay_up/1 -> OR/2
  OR/1 -> switch2/2
  delay_down/1 -> switch2/3

== system gm_smartCart4_1_work/head/Reciver/Unit Delay Enabled Resettable15 ==
  data_in : Inport
  Enb : Inport  Port=2
  Reset : Inport  Port=3
  Const_Zero : Constant  Value=0  OutDataTypeStr=boolean
  Initial_Condition : Constant  Value=0.0  OutDataTypeStr=Inherit: Inherit via back propagation
  OR : Logic  Operator=OR
  delay_down : UnitDelay  SampleTime=-1
  delay_up : UnitDelay  InitialCondition=1  SampleTime=-1
  switch0 : Switch  SaturateOnIntegerOverflow=on  InputSameDT=on
  switch1 : Switch  SaturateOnIntegerOverflow=on  InputSameDT=on
  switch2 : Switch  SaturateOnIntegerOverflow=on  InputSameDT=on
  data_out : Outport
  wires:
  data_in/1 -> switch0/1
  Enb/1 -> switch0/2
  switch2/1 -> switch0/3, data_out/1
  Initial_Condition/1 -> switch1/1, switch2/1
  Reset/1 -> switch1/2, OR/1
  switch0/1 -> switch1/3
  Const_Zero/1 -> delay_up/1
  switch1/1 -> delay_down/1
  delay_up/1 -> OR/2
  OR/1 -> switch2/2
  delay_down/1 -> switch2/3

== system gm_smartCart4_1_work/head/Reciver/Unit Delay Enabled Resettable16 ==
  data_in : Inport
  Enb : Inport  Port=2
  Reset : Inport  Port=3
  Const_Zero : Constant  Value=0  OutDataTypeStr=boolean
  Initial_Condition : Constant  Value=0.0  OutDataTypeStr=Inherit: Inherit via back propagation
  OR : Logic  Operator=OR
  delay_down : UnitDelay  SampleTime=-1
  delay_up : UnitDelay  InitialCondition=1  SampleTime=-1
  switch0 : Switch  SaturateOnIntegerOverflow=on  InputSameDT=on
  switch1 : Switch  SaturateOnIntegerOverflow=on  InputSameDT=on
  switch2 : Switch  SaturateOnIntegerOverflow=on  InputSameDT=on
  data_out : Outport
  wires:
  data_in/1 -> switch0/1
  Enb/1 -> switch0/2
  switch2/1 -> switch0/3, data_out/1
  Initial_Condition/1 -> switch1/1, switch2/1
  Reset/1 -> switch1/2, OR/1
  switch0/1 -> switch1/3
  Const_Zero/1 -> delay_up/1
  switch1/1 -> delay_down/1
  delay_up/1 -> OR/2
  OR/1 -> switch2/2
  delay_down/1 -> switch2/3

== system gm_smartCart4_1_work/head/Reciver/Unit Delay Enabled Resettable17 ==
  data_in : Inport
  Enb : Inport  Port=2
  Reset : Inport  Port=3
  Const_Zero : Constant  Value=0  OutDataTypeStr=boolean
  Initial_Condition : Constant  Value=0.0  OutDataTypeStr=Inherit: Inherit via back propagation
  OR : Logic  Operator=OR
  delay_down : UnitDelay  SampleTime=-1
  delay_up : UnitDelay  InitialCondition=1  SampleTime=-1
  switch0 : Switch  SaturateOnIntegerOverflow=on  InputSameDT=on
  switch1 : Switch  SaturateOnIntegerOverflow=on  InputSameDT=on
  switch2 : Switch  SaturateOnIntegerOverflow=on  InputSameDT=on
  data_out : Outport
  wires:
  data_in/1 -> switch0/1
  Enb/1 -> switch0/2
  switch2/1 -> switch0/3, data_out/1
  Initial_Condition/1 -> switch1/1, switch2/1
  Reset/1 -> switch1/2, OR/1
  switch0/1 -> switch1/3
  Const_Zero/1 -> delay_up/1
  switch1/1 -> delay_down/1
  delay_up/1 -> OR/2
  OR/1 -> switch2/2
  delay_down/1 -> switch2/3

== system gm_smartCart4_1_work/head/Reciver/Unit Delay Enabled Resettable18 ==
  data_in : Inport
  Enb : Inport  Port=2
  Reset : Inport  Port=3
  Const_Zero : Constant  Value=0  OutDataTypeStr=boolean
  Initial_Condition : Constant  Value=0.0  OutDataTypeStr=Inherit: Inherit via back propagation
  OR : Logic  Operator=OR
  delay_down : UnitDelay  SampleTime=-1
  delay_up : UnitDelay  InitialCondition=1  SampleTime=-1
  switch0 : Switch  SaturateOnIntegerOverflow=on  InputSameDT=on
  switch1 : Switch  SaturateOnIntegerOverflow=on  InputSameDT=on
  switch2 : Switch  SaturateOnIntegerOverflow=on  InputSameDT=on
  data_out : Outport
  wires:
  data_in/1 -> switch0/1
  Enb/1 -> switch0/2
  switch2/1 -> switch0/3, data_out/1
  Initial_Condition/1 -> switch1/1, switch2/1
  Reset/1 -> switch1/2, OR/1
  switch0/1 -> switch1/3
  Const_Zero/1 -> delay_up/1
  switch1/1 -> delay_down/1
  delay_up/1 -> OR/2
  OR/1 -> switch2/2
  delay_down/1 -> switch2/3

== system gm_smartCart4_1_work/head/Reciver/Unit Delay Enabled Resettable19 ==
  data_in : Inport
  Enb : Inport  Port=2
  Reset : Inport  Port=3
  Const_Zero : Constant  Value=0  OutDataTypeStr=boolean
  Initial_Condition : Constant  Value=0.0  OutDataTypeStr=Inherit: Inherit via back propagation
  OR : Logic  Operator=OR
  delay_down : UnitDelay  SampleTime=-1
  delay_up : UnitDelay  InitialCondition=1  SampleTime=-1
  switch0 : Switch  SaturateOnIntegerOverflow=on  InputSameDT=on
  switch1 : Switch  SaturateOnIntegerOverflow=on  InputSameDT=on
  switch2 : Switch  SaturateOnIntegerOverflow=on  InputSameDT=on
  data_out : Outport
  wires:
  data_in/1 -> switch0/1
  Enb/1 -> switch0/2
  switch2/1 -> switch0/3, data_out/1
  Initial_Condition/1 -> switch1/1, switch2/1
  Reset/1 -> switch1/2, OR/1
  switch0/1 -> switch1/3
  Const_Zero/1 -> delay_up/1
  switch1/1 -> delay_down/1
  delay_up/1 -> OR/2
  OR/1 -> switch2/2
  delay_down/1 -> switch2/3

== system gm_smartCart4_1_work/head/Reciver/Unit Delay Enabled Resettable2 ==
  data_in : Inport
  Enb : Inport  Port=2
  Reset : Inport  Port=3
  Const_Zero : Constant  Value=0  OutDataTypeStr=boolean
  Initial_Condition : Constant  Value=0.0  OutDataTypeStr=Inherit: Inherit via back propagation
  OR : Logic  Operator=OR
  delay_down : UnitDelay  SampleTime=-1
  delay_up : UnitDelay  InitialCondition=1  SampleTime=-1
  switch0 : Switch  SaturateOnIntegerOverflow=on  InputSameDT=on
  switch1 : Switch  SaturateOnIntegerOverflow=on  InputSameDT=on
  switch2 : Switch  SaturateOnIntegerOverflow=on  InputSameDT=on
  data_out : Outport
  wires:
  data_in/1 -> switch0/1
  Enb/1 -> switch0/2
  switch2/1 -> switch0/3, data_out/1
  Initial_Condition/1 -> switch1/1, switch2/1
  Reset/1 -> switch1/2, OR/1
  switch0/1 -> switch1/3
  Const_Zero/1 -> delay_up/1
  switch1/1 -> delay_down/1
  delay_up/1 -> OR/2
  OR/1 -> switch2/2
  delay_down/1 -> switch2/3

== system gm_smartCart4_1_work/head/Reciver/Unit Delay Enabled Resettable3 ==
  data_in : Inport
  Enb : Inport  Port=2
  Reset : Inport  Port=3
  Const_Zero : Constant  Value=0  OutDataTypeStr=boolean
  Initial_Condition : Constant  Value=0.0  OutDataTypeStr=Inherit: Inherit via back propagation
  OR : Logic  Operator=OR
  delay_down : UnitDelay  SampleTime=-1
  delay_up : UnitDelay  InitialCondition=1  SampleTime=-1
  switch0 : Switch  SaturateOnIntegerOverflow=on  InputSameDT=on
  switch1 : Switch  SaturateOnIntegerOverflow=on  InputSameDT=on
  switch2 : Switch  SaturateOnIntegerOverflow=on  InputSameDT=on
  data_out : Outport
  wires:
  data_in/1 -> switch0/1
  Enb/1 -> switch0/2
  switch2/1 -> switch0/3, data_out/1
  Initial_Condition/1 -> switch1/1, switch2/1
  Reset/1 -> switch1/2, OR/1
  switch0/1 -> switch1/3
  Const_Zero/1 -> delay_up/1
  switch1/1 -> delay_down/1
  delay_up/1 -> OR/2
  OR/1 -> switch2/2
  delay_down/1 -> switch2/3

== system gm_smartCart4_1_work/head/Reciver/Unit Delay Enabled Resettable4 ==
  data_in : Inport
  Enb : Inport  Port=2
  Reset : Inport  Port=3
  Const_Zero : Constant  Value=0  OutDataTypeStr=boolean
  Initial_Condition : Constant  Value=0.0  OutDataTypeStr=Inherit: Inherit via back propagation
  OR : Logic  Operator=OR
  delay_down : UnitDelay  SampleTime=-1
  delay_up : UnitDelay  InitialCondition=1  SampleTime=-1
  switch0 : Switch  SaturateOnIntegerOverflow=on  InputSameDT=on
  switch1 : Switch  SaturateOnIntegerOverflow=on  InputSameDT=on
  switch2 : Switch  SaturateOnIntegerOverflow=on  InputSameDT=on
  data_out : Outport
  wires:
  data_in/1 -> switch0/1
  Enb/1 -> switch0/2
  switch2/1 -> switch0/3, data_out/1
  Initial_Condition/1 -> switch1/1, switch2/1
  Reset/1 -> switch1/2, OR/1
  switch0/1 -> switch1/3
  Const_Zero/1 -> delay_up/1
  switch1/1 -> delay_down/1
  delay_up/1 -> OR/2
  OR/1 -> switch2/2
  delay_down/1 -> switch2/3

== system gm_smartCart4_1_work/head/Reciver/Unit Delay Enabled Resettable5 ==
  data_in : Inport
  Enb : Inport  Port=2
  Reset : Inport  Port=3
  Const_Zero : Constant  Value=0  OutDataTypeStr=boolean
  Initial_Condition : Constant  Value=0.0  OutDataTypeStr=Inherit: Inherit via back propagation
  OR : Logic  Operator=OR
  delay_down : UnitDelay  SampleTime=-1
  delay_up : UnitDelay  InitialCondition=1  SampleTime=-1
  switch0 : Switch  SaturateOnIntegerOverflow=on  InputSameDT=on
  switch1 : Switch  SaturateOnIntegerOverflow=on  InputSameDT=on
  switch2 : Switch  SaturateOnIntegerOverflow=on  InputSameDT=on
  data_out : Outport
  wires:
  data_in/1 -> switch0/1
  Enb/1 -> switch0/2
  switch2/1 -> switch0/3, data_out/1
  Initial_Condition/1 -> switch1/1, switch2/1
  Reset/1 -> switch1/2, OR/1
  switch0/1 -> switch1/3
  Const_Zero/1 -> delay_up/1
  switch1/1 -> delay_down/1
  delay_up/1 -> OR/2
  OR/1 -> switch2/2
  delay_down/1 -> switch2/3

== system gm_smartCart4_1_work/head/Reciver/Unit Delay Enabled Resettable6 ==
  data_in : Inport
  Enb : Inport  Port=2
  Reset : Inport  Port=3
  Const_Zero : Constant  Value=0  OutDataTypeStr=boolean
  Initial_Condition : Constant  Value=0.0  OutDataTypeStr=Inherit: Inherit via back propagation
  OR : Logic  Operator=OR
  delay_down : UnitDelay  SampleTime=-1
  delay_up : UnitDelay  InitialCondition=1  SampleTime=-1
  switch0 : Switch  SaturateOnIntegerOverflow=on  InputSameDT=on
  switch1 : Switch  SaturateOnIntegerOverflow=on  InputSameDT=on
  switch2 : Switch  SaturateOnIntegerOverflow=on  InputSameDT=on
  data_out : Outport
  wires:
  data_in/1 -> switch0/1
  Enb/1 -> switch0/2
  switch2/1 -> switch0/3, data_out/1
  Initial_Condition/1 -> switch1/1, switch2/1
  Reset/1 -> switch1/2, OR/1
  switch0/1 -> switch1/3
  Const_Zero/1 -> delay_up/1
  switch1/1 -> delay_down/1
  delay_up/1 -> OR/2
  OR/1 -> switch2/2
  delay_down/1 -> switch2/3

== system gm_smartCart4_1_work/head/Reciver/Unit Delay Enabled Resettable7 ==
  data_in : Inport
  Enb : Inport  Port=2
  Reset : Inport  Port=3
  Const_Zero : Constant  Value=0  OutDataTypeStr=boolean
  Initial_Condition : Constant  Value=0.0  OutDataTypeStr=Inherit: Inherit via back propagation
  OR : Logic  Operator=OR
  delay_down : UnitDelay  SampleTime=-1
  delay_up : UnitDelay  InitialCondition=1  SampleTime=-1
  switch0 : Switch  SaturateOnIntegerOverflow=on  InputSameDT=on
  switch1 : Switch  SaturateOnIntegerOverflow=on  InputSameDT=on
  switch2 : Switch  SaturateOnIntegerOverflow=on  InputSameDT=on
  data_out : Outport
  wires:
  data_in/1 -> switch0/1
  Enb/1 -> switch0/2
  switch2/1 -> switch0/3, data_out/1
  Initial_Condition/1 -> switch1/1, switch2/1
  Reset/1 -> switch1/2, OR/1
  switch0/1 -> switch1/3
  Const_Zero/1 -> delay_up/1
  switch1/1 -> delay_down/1
  delay_up/1 -> OR/2
  OR/1 -> switch2/2
  delay_down/1 -> switch2/3

== system gm_smartCart4_1_work/head/Reciver/Unit Delay Enabled Resettable8 ==
  data_in : Inport
  Enb : Inport  Port=2
  Reset : Inport  Port=3
  Const_Zero : Constant  Value=0  OutDataTypeStr=boolean
  Initial_Condition : Constant  Value=0.0  OutDataTypeStr=Inherit: Inherit via back propagation
  OR : Logic  Operator=OR
  delay_down : UnitDelay  SampleTime=-1
  delay_up : UnitDelay  InitialCondition=1  SampleTime=-1
  switch0 : Switch  SaturateOnIntegerOverflow=on  InputSameDT=on
  switch1 : Switch  SaturateOnIntegerOverflow=on  InputSameDT=on
  switch2 : Switch  SaturateOnIntegerOverflow=on  InputSameDT=on
  data_out : Outport
  wires:
  data_in/1 -> switch0/1
  Enb/1 -> switch0/2
  switch2/1 -> switch0/3, data_out/1
  Initial_Condition/1 -> switch1/1, switch2/1
  Reset/1 -> switch1/2, OR/1
  switch0/1 -> switch1/3
  Const_Zero/1 -> delay_up/1
  switch1/1 -> delay_down/1
  delay_up/1 -> OR/2
  OR/1 -> switch2/2
  delay_down/1 -> switch2/3

== system gm_smartCart4_1_work/head/Reciver/Unit Delay Enabled Resettable9 ==
  data_in : Inport
  Enb : Inport  Port=2
  Reset : Inport  Port=3
  Const_Zero : Constant  Value=0  OutDataTypeStr=boolean
  Initial_Condition : Constant  Value=0.0  OutDataTypeStr=Inherit: Inherit via back propagation
  OR : Logic  Operator=OR
  delay_down : UnitDelay  SampleTime=-1
  delay_up : UnitDelay  InitialCondition=1  SampleTime=-1
  switch0 : Switch  SaturateOnIntegerOverflow=on  InputSameDT=on
  switch1 : Switch  SaturateOnIntegerOverflow=on  InputSameDT=on
  switch2 : Switch  SaturateOnIntegerOverflow=on  InputSameDT=on
  data_out : Outport
  wires:
  data_in/1 -> switch0/1
  Enb/1 -> switch0/2
  switch2/1 -> switch0/3, data_out/1
  Initial_Condition/1 -> switch1/1, switch2/1
  Reset/1 -> switch1/2, OR/1
  switch0/1 -> switch1/3
  Const_Zero/1 -> delay_up/1
  switch1/1 -> delay_down/1
  delay_up/1 -> OR/2
  OR/1 -> switch2/2
  delay_down/1 -> switch2/3

== system gm_smartCart4_1_work/head/Reciver/signal_edg ==
  In1 : Inport  OutDataTypeStr=boolean  SampleTime=1
  Delay4 : Delay  DelayLength=1  InitialCondition=0
  Logical Operator1 : Logic  Operator=XOR  AllPortsSameDT=off  OutDataTypeStr=boolean
  Logical Operator15 : Logic  AllPortsSameDT=off  OutDataTypeStr=boolean
  Out1 : Outport  OutDataTypeStr=boolean
  wires:
  Logical Operator15/1 -> Out1/1
  Logical Operator1/1 -> Logical Operator15/1
  Delay4/1 -> Logical Operator1/1
  In1/1 -> Delay4/1, Logical Operator1/2, Logical Operator15/2

== system gm_smartCart4_1_work/head/Reciver/signal_edg5 ==
  In1 : Inport  OutDataTypeStr=boolean  SampleTime=1
  Delay4 : Delay  DelayLength=1  InitialCondition=0
  Logical Operator1 : Logic  Operator=XOR  AllPortsSameDT=off  OutDataTypeStr=boolean
  Logical Operator15 : Logic  AllPortsSameDT=off  OutDataTypeStr=boolean
  Out1 : Outport  OutDataTypeStr=boolean
  wires:
  Logical Operator15/1 -> Out1/1
  Logical Operator1/1 -> Logical Operator15/1
  Delay4/1 -> Logical Operator1/1
  In1/1 -> Delay4/1, Logical Operator1/2, Logical Operator15/2

== system gm_smartCart4_1_work/head/Transmit/latch_data ==
  data_in : Inport
  Enb : Inport  Port=2
  Reset : Inport  Port=3
  Const_Zero : Constant  Value=0  OutDataTypeStr=boolean
  Initial_Condition : Constant  Value=0  OutDataTypeStr=Inherit: Inherit via back propagation
  OR : Logic  Operator=OR
  delay_down : UnitDelay  SampleTime=-1
  delay_up : UnitDelay  InitialCondition=1  SampleTime=-1
  switch0 : Switch  SaturateOnIntegerOverflow=on  InputSameDT=on
  switch1 : Switch  SaturateOnIntegerOverflow=on  InputSameDT=on
  switch2 : Switch  SaturateOnIntegerOverflow=on  InputSameDT=on
  data_out : Outport
  wires:
  data_in/1 -> switch0/1
  Enb/1 -> switch0/2
  switch2/1 -> switch0/3, data_out/1
  Initial_Condition/1 -> switch1/1, switch2/1
  Reset/1 -> switch1/2, OR/1
  switch0/1 -> switch1/3
  Const_Zero/1 -> delay_up/1
  switch1/1 -> delay_down/1
  delay_up/1 -> OR/2
  OR/1 -> switch2/2
  delay_down/1 -> switch2/3
